simulink library "csc_apc_actionpoint_collection_lib"  (R2015b)
settings: Solver=VariableStepAuto  StartTime=0.0  StopTime=10.0  RelTol=1e-3
libraries: csc_eap_evaluate_ap_lib x8, util_info_lib x1
settings Model: Creator=Mark Agbayani  LastModifiedBy=jimkaidy

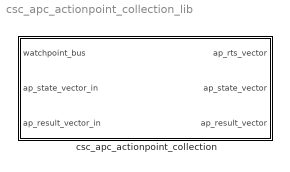
== system csc_apc_actionpoint_collection_lib ==
  csc_apc_actionpoint_collection : Subsystem
      mask Display: color('blue');text(0.05, 0.02, 'MoonEx', 'HorizontalAlignment', 'Left', 'VerticalAlignment', 'Bottom');color('red');text(0.95, 0.02, 'Autogenerated', 'HorizontalAlignment', 'Right', 'VerticalAlignment', 'Bottom');

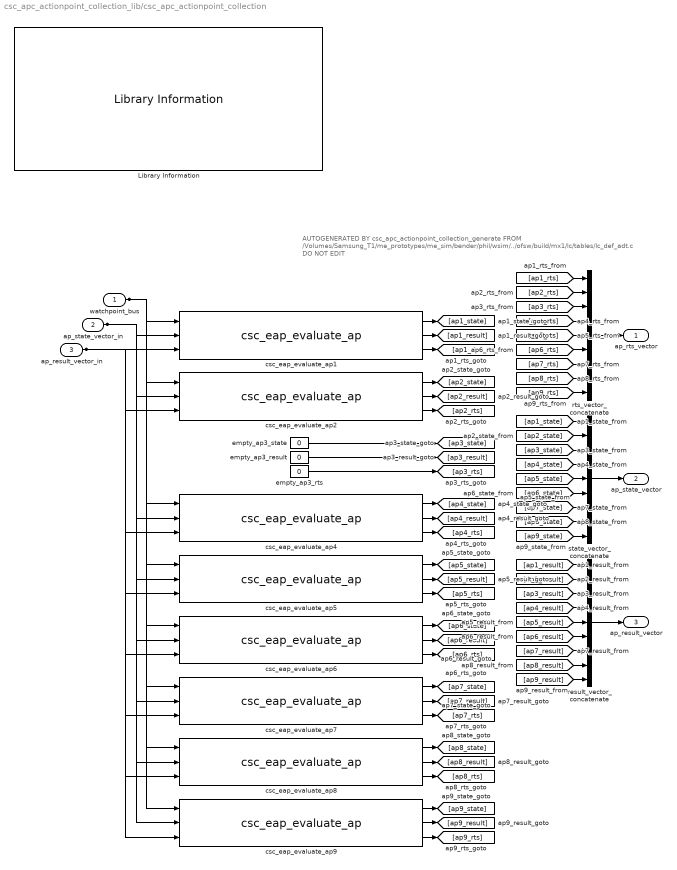
== system csc_apc_actionpoint_collection_lib/csc_apc_actionpoint_collection ==
  note: AUTOGENERATED BY csc_apc_actionpoint_collection_generate FROM
      | /Volumes/Samsung_T1/me_prototypes/me_sim/bender/phil/wsim/../ofsw/build/mx1/lc/tables/lc_def_adt.c
      | DO NOT EDIT
  watchpoint_bus : Inport
  ap_state_vector_in : Inport  Port=2
  ap_result_vector_in : Inport  Port=3
  Library Information : util_info_lib/Library Information  owner='escrane'
  csc_eap_evaluate_ap1 : csc_eap_evaluate_ap_lib/csc_eap_evaluate_ap  ap_id=1  ap_start_rts_id=1  ap_max_fail_before_rts=1  ap_wp_equation=1  ap_default_state=DISABLED  ap_event_type=INFORMATION  ap_event_id=21  ap_event_text=Executing startup RTS...
  csc_eap_evaluate_ap2 : csc_eap_evaluate_ap_lib/csc_eap_evaluate_ap  ap_id=2  ap_start_rts_id=10  ap_max_fail_before_rts=1  ap_wp_equation=4  ap_default_state=ACTIVE  ap_event_type=INFORMATION  ap_event_id=22  ap_event_text=Transition to Approach Targeting
  csc_eap_evaluate_ap4 : csc_eap_evaluate_ap_lib/csc_eap_evaluate_ap  ap_id=4  ap_start_rts_id=12  ap_max_fail_before_rts=1  ap_wp_equation=4 5 AND  ap_default_state=ACTIVE  ap_event_type=INFORMATION  ap_event_id=24  ap_event_text=Transition to Terminal Descent
  csc_eap_evaluate_ap5 : csc_eap_evaluate_ap_lib/csc_eap_evaluate_ap  ap_id=5  ap_start_rts_id=13  ap_max_fail_before_rts=1  ap_wp_equation=2 3 AND 7 AND 8 NOT AND  ap_default_state=ACTIVE  ap_event_type=INFORMATION  ap_event_id=25  ap_event_text=Transition to surface mode!
  csc_eap_evaluate_ap6 : csc_eap_evaluate_ap_lib/csc_eap_evaluate_ap  ap_id=6  ap_start_rts_id=14  ap_max_fail_before_rts=1  ap_wp_equation=9  ap_default_state=ACTIVE  ap_event_type=INFORMATION  ap_event_id=26  ap_event_text=Main Engine Fire! -> Coarse Pitch/Yaw, Vernier Roll
  csc_eap_evaluate_ap7 : csc_eap_evaluate_ap_lib/csc_eap_evaluate_ap  ap_id=7  ap_start_rts_id=15  ap_max_fail_before_rts=1  ap_wp_equation=10 3 NOT AND 6 NOT AND  ap_default_state=PASSIVE  ap_event_type=INFORMATION  ap_event_id=27  ap_event_text=Coast in Vernier ACS
  csc_eap_evaluate_ap8 : csc_eap_evaluate_ap_lib/csc_eap_evaluate_ap  ap_id=8  ap_start_rts_id=18  ap_max_fail_before_rts=1  ap_wp_equation=3 9 NOT AND  ap_default_state=ACTIVE  ap_event_type=INFORMATION  ap_event_id=28  ap_event_text=Terminal, Coarse Pitch/Yaw, Vernier Roll ACS
  csc_eap_evaluate_ap9 : csc_eap_evaluate_ap_lib/csc_eap_evaluate_ap  ap_id=9  ap_start_rts_id=17  ap_max_fail_before_rts=1  ap_wp_equation=14 12 AND 13 NOT AND 11 NOT AND 6 NOT AND 3 NOT AND  ap_default_state=ACTIVE  ap_event_type=INFORMATION  ap_event_id=29  ap_event_text=Landing Hold
  empty_ap3_result : Constant  Value=0  OutDataTypeStr=boolean
  empty_ap3_rts : Constant  Value=0  OutDataTypeStr=uint16
  empty_ap3_state : Constant  Value=0  OutDataTypeStr=uint8
  result_vector_concatenate : Concatenate  NumInputs=9
  rts_vector_concatenate : Concatenate  NumInputs=9
  state_vector_concatenate : Concatenate  NumInputs=9
  ap_rts_vector : Outport
  ap_state_vector : Outport  Port=2
  ap_result_vector : Outport  Port=3
  wires:
  rts_vector_concatenate/1 -> ap_rts_vector/1
  state_vector_concatenate/1 -> ap_state_vector/1
  result_vector_concatenate/1 -> ap_result_vector/1
  [ap1_rts] -> rts_vector_concatenate/1
  [ap1_state] -> state_vector_concatenate/1
  [ap1_result] -> result_vector_concatenate/1
  ap_result_vector_in/1 -> csc_eap_evaluate_ap1/3, csc_eap_evaluate_ap2/3, csc_eap_evaluate_ap4/3, csc_eap_evaluate_ap5/3, csc_eap_evaluate_ap6/3, csc_eap_evaluate_ap7/3, csc_eap_evaluate_ap8/3, csc_eap_evaluate_ap9/3
  ap_state_vector_in/1 -> csc_eap_evaluate_ap1/2, csc_eap_evaluate_ap2/2, csc_eap_evaluate_ap4/2, csc_eap_evaluate_ap5/2, csc_eap_evaluate_ap6/2, csc_eap_evaluate_ap7/2, csc_eap_evaluate_ap8/2, csc_eap_evaluate_ap9/2
  watchpoint_bus/1 -> csc_eap_evaluate_ap1/1, csc_eap_evaluate_ap2/1, csc_eap_evaluate_ap4/1, csc_eap_evaluate_ap5/1, csc_eap_evaluate_ap6/1, csc_eap_evaluate_ap7/1, csc_eap_evaluate_ap8/1, csc_eap_evaluate_ap9/1
  csc_eap_evaluate_ap1/1 -> [ap1_state]
  csc_eap_evaluate_ap1/2 -> [ap1_result]
  csc_eap_evaluate_ap1/3 -> [ap1_rts]
  [ap2_rts] -> rts_vector_concatenate/2
  [ap2_state] -> state_vector_concatenate/2
  [ap2_result] -> result_vector_concatenate/2
  csc_eap_evaluate_ap2/1 -> [ap2_state]
  csc_eap_evaluate_ap2/2 -> [ap2_result]
  csc_eap_evaluate_ap2/3 -> [ap2_rts]
  [ap3_rts] -> rts_vector_concatenate/3
  [ap3_state] -> state_vector_concatenate/3
  [ap3_result] -> result_vector_concatenate/3
  empty_ap3_state/1 -> [ap3_state]
  empty_ap3_result/1 -> [ap3_result]
  empty_ap3_rts/1 -> [ap3_rts]
  [ap4_rts] -> rts_vector_concatenate/4
  [ap4_state] -> state_vector_concatenate/4
  [ap4_result] -> result_vector_concatenate/4
  csc_eap_evaluate_ap4/1 -> [ap4_state]
  csc_eap_evaluate_ap4/2 -> [ap4_result]
  csc_eap_evaluate_ap4/3 -> [ap4_rts]
  [ap5_rts] -> rts_vector_concatenate/5
  [ap5_state] -> state_vector_concatenate/5
  [ap5_result] -> result_vector_concatenate/5
  csc_eap_evaluate_ap5/1 -> [ap5_state]
  csc_eap_evaluate_ap5/2 -> [ap5_result]
  csc_eap_evaluate_ap5/3 -> [ap5_rts]
  [ap6_rts] -> rts_vector_concatenate/6
  [ap6_state] -> state_vector_concatenate/6
  [ap6_result] -> result_vector_concatenate/6
  csc_eap_evaluate_ap6/1 -> [ap6_state]
  csc_eap_evaluate_ap6/2 -> [ap6_result]
  csc_eap_evaluate_ap6/3 -> [ap6_rts]
  [ap7_rts] -> rts_vector_concatenate/7
  [ap7_state] -> state_vector_concatenate/7
  [ap7_result] -> result_vector_concatenate/7
  csc_eap_evaluate_ap7/1 -> [ap7_state]
  csc_eap_evaluate_ap7/2 -> [ap7_result]
  csc_eap_evaluate_ap7/3 -> [ap7_rts]
  [ap8_rts] -> rts_vector_concatenate/8
  [ap8_state] -> state_vector_concatenate/8
  [ap8_result] -> result_vector_concatenate/8
  csc_eap_evaluate_ap8/1 -> [ap8_state]
  csc_eap_evaluate_ap8/2 -> [ap8_result]
  csc_eap_evaluate_ap8/3 -> [ap8_rts]
  [ap9_rts] -> rts_vector_concatenate/9
  [ap9_state] -> state_vector_concatenate/9
  [ap9_result] -> result_vector_concatenate/9
  csc_eap_evaluate_ap9/1 -> [ap9_state]
  csc_eap_evaluate_ap9/2 -> [ap9_result]
  csc_eap_evaluate_ap9/3 -> [ap9_rts]
